simulink model "SizingFlightModel"  (R2024b)
settings: Solver=VariableStepAuto  StartTime=0.0  StopTime=50  RelTol=1e-3
values from neighbouring files (symbols this model uses):
  gamma = 1.4    [PotentialOrificeSize.m]    (also in runSizingSim.m = 1.23; sizingSweep.m = 1.23)
  isp = 215    [runSizingSim.m]    (also in sizingSweep.m)
  M = readmatrix(filename, 'NumHeaderLines', 1)    [STEPFNC_ODE_THRUST.m]    (also in runSizingSim.m = 0.0288; sizingSweep.m = 0.0288)
  m_0 = m_payload + 1.15 * m_fuel    (= 25.75)    [runSizingSim.m]    (also in sizingSweep.m = m_payload + 1.15 * m_fuel)
  m_fuel = 5.0    (= 5)    [runSizingSim.m]
  mdot = mdot_limit    (= 0.4)    [PotentialOrificeSize.m]    (also in runSizingSim.m = 0.359302325581; sizingSweep.m = result_table.MassFlowRate_kgps)
  p_c = 520 * 6894.76    (= 3585275.2)    [runSizingSim.m]    (also in sizingSweep.m)
  r = 0.08    [runSizingSim.m]    (also in sizingPrep.m = 0.1016; sizingSweep.m; tankEquilibrium.m = 0.1016)
  T_c = 3200    [runSizingSim.m]    (also in sizingSweep.m)
libraries: simulink x2, aerolibatmos2 x2
settings Model: Creator=Nicholas Quillin  LastModifiedBy=Nicholas Quillin

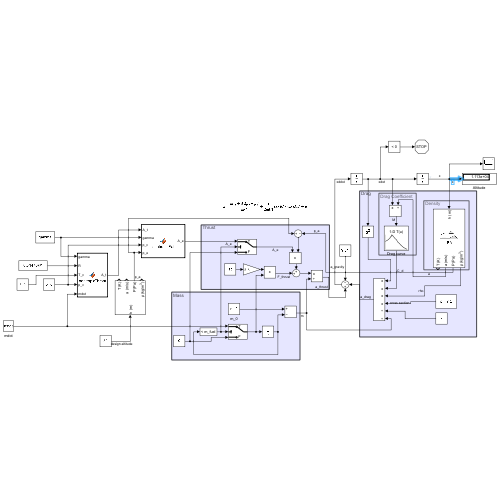
[thumbnail: Simulink's stored preview of the top-level diagram]
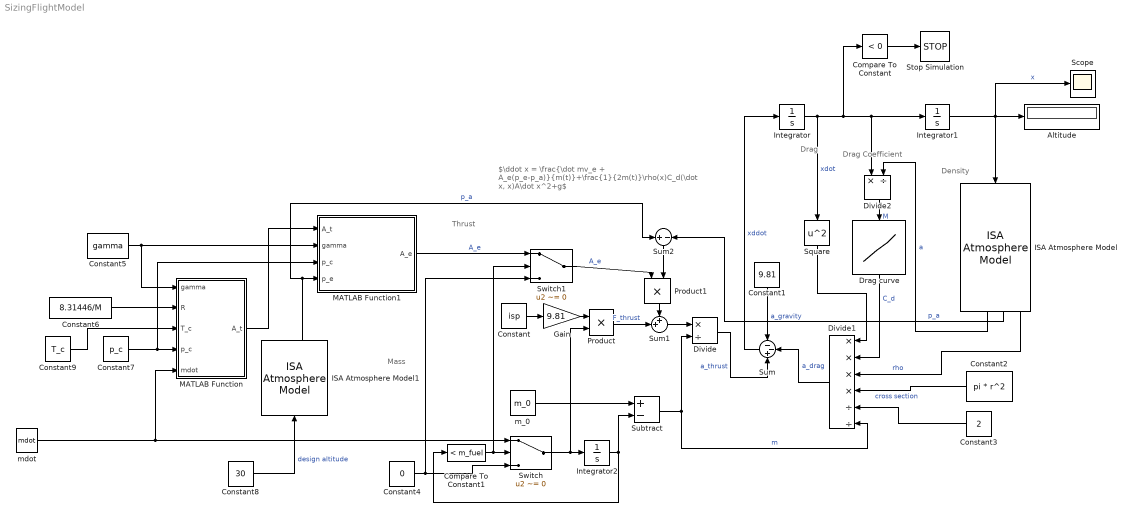
== system SizingFlightModel ==
  note: $\ddot x = \frac{\dot mv_e + A_e(p_e-p_a)}{m(t)}+\frac{1}{2m(t)}\rho(x)C_d(\dot x, x)A\dot x^2+g$
  note: Density
  note: Drag Coefficient
  note: Mass
  note: Thrust
  note: Drag
  Altitude : Display
  Compare To Constant : simulink/Logic and Bit Operations/Compare To Constant  relop=<  const=0  OutDataTypeStr=boolean
  Compare To Constant1 : simulink/Logic and Bit Operations/Compare To Constant  relop=<  const=m_fuel  OutDataTypeStr=boolean
  Constant : Constant  Value=isp
  Constant1 : Constant  Value=9.81
  Constant2 : Constant  Value=pi * r^2
  Constant3 : Constant  Value=2
  Constant4 : Constant  Value=0
  Constant5 : Constant  Value=gamma
  Constant6 : Constant  Value=8.31446/M
  Constant7 : Constant  Value=p_c
  Constant8 : Constant  Value=30
  Constant9 : Constant  Value=T_c
  Divide : Product  Inputs=*/
  Divide1 : Product  Inputs=****//
  Divide2 : Product  Inputs=*/
  Drag curve : Lookup_n-D  NumberOfTableDimensions=1  BreakpointsForDimension1=[0.2 0.4 0.6 0.8 0.9 0.975 1.0 1.025 1.05 1.1 1.2 1.4 1.6 1.8 2.0 2.2 2.4 2.6 2.8 3.0]  Table=[0.52 0.534 0.559 0.592 0.612 0.628 0.649 0.651 0.655 0.648 0.629 0.590 0.549 0.508 0.472 0.442 0.414 0.390 0.371 0.355]  InterpMethod=Linear Lagrange  InternalRulePriority=Speed  RndMeth=Simplest
  Gain : Gain  Gain=9.81
  ISA Atmosphere Model : aerolibatmos2/ISA Atmosphere Model  useExtended=off  action=Warning  custom=off  viscosityOut=off  g=9.80665  gamma=1.4  R=287.0531  L=0.0065  h_trop=11000  h_strat=20000  rho0=1.225  P0=101325  T0=288.15  h0=0  S=110.4  Tref=273.15  muref=1.716e-5
  ISA Atmosphere Model1 : aerolibatmos2/ISA Atmosphere Model  useExtended=off  action=Warning  custom=off  viscosityOut=off  g=9.80665  gamma=1.4  R=287.0531  L=0.0065  h_trop=11000  h_strat=20000  rho0=1.225  P0=101325  T0=288.15  h0=0  S=110.4  Tref=273.15  muref=1.716e-5
  Integrator : Integrator
  Integrator1 : Integrator
  Integrator2 : Integrator
  MATLAB Function : MATLAB Function  TreatAsAtomicUnit=on
  MATLAB Function1 : MATLAB Function  TreatAsAtomicUnit=on
  Product : Product
  Product1 : Product
  Scope : Scope
  Square : Math  Operator=square
  Stop Simulation : Stop
  Subtract : Sum  Inputs=+-
  Sum : Sum  Inputs=--+
  Sum1 : Sum  Inputs=++|
  Sum2 : Sum  Inputs=+-
  Switch : Switch  Criteria=u2 ~= 0  Threshold=m_fuel  SaturateOnIntegerOverflow=off  InputSameDT=off
  Switch1 : Switch  Criteria=u2 ~= 0  Threshold=m_fuel  SaturateOnIntegerOverflow=off  InputSameDT=off
  m_0 : Constant  Value=m_0
  mdot : Constant  Value=mdot
  wires:
  Sum/1 -> Integrator/1  "xddot"
  Integrator/1 -> Square/1, Compare To Constant/1, Divide2/1, Integrator1/1  "xdot"
  Integrator1/1 -> Altitude/1, Scope/1, ISA Atmosphere Model/1  "x"
  m_0/1 -> Subtract/1
  Integrator2/1 -> Subtract/2, Compare To Constant1/1
  Subtract/1 -> Divide1/6, Divide/2  "m"
  Drag curve/1 -> Divide1/2  "C_d"
  Switch/1 -> Product/2, Integrator2/1
  mdot/1 -> MATLAB Function/5(mdot), Switch/1
  Divide/1 -> Sum/3  "a_thrust"
  Divide1/1 -> Sum/2  "a_drag"
  Constant1/1 -> Sum/1  "a_gravity"
  Square/1 -> Divide1/1
  ISA Atmosphere Model/4 -> Divide1/3  "rho"
  Constant2/1 -> Divide1/4  "cross section"
  Constant3/1 -> Divide1/5
  Divide2/1 -> Drag curve/1  "M"
  ISA Atmosphere Model/2 -> Divide2/2  "a"
  Compare To Constant/1 -> Stop Simulation/1
  Compare To Constant1/1 -> Switch1/2, Switch/2
  Constant4/1 -> Switch1/3, Switch/3
  MATLAB Function1/1(A_e) -> Switch1/1  "A_e"
  Product/1 -> Sum1/2  "F_thrust"
  Sum1/1 -> Divide/1
  Product1/1 -> Sum1/1
  Switch1/1 -> Product1/1  "A_e"
  Sum2/1 -> Product1/2
  ISA Atmosphere Model/3 -> Sum2/2  "p_a"
  Constant/1 -> Gain/1
  Gain/1 -> Product/1
  MATLAB Function/1(A_t) -> MATLAB Function1/1(A_t)
  Constant7/1 -> MATLAB Function1/3(p_c), MATLAB Function/4(p_c)
  ISA Atmosphere Model1/3 -> Sum2/1, MATLAB Function1/4(p_e)  "p_a"
  Constant5/1 -> MATLAB Function/1(gamma), MATLAB Function1/2(gamma)
  Constant6/1 -> MATLAB Function/2(R)
  Constant8/1 -> ISA Atmosphere Model1/1  "design altitude"
  Constant9/1 -> MATLAB Function/3(T_c)

== matlab function SizingFlightModel/MATLAB Function1 ==
  data: A_t input; gamma input; A_e output; p_c input; p_e input
function A_e = isentropicExit(A_t, gamma, p_c, p_e)
A_e = A_t * (2/(gamma+1))^(1/(gamma-1)) * (p_c/p_e)^(1/gamma)...
    * sqrt(((gamma-1)/(gamma+1)*(1-(p_e/p_c)^((gamma-1)/gamma)))^-1)

== matlab function SizingFlightModel/MATLAB Function ==
  data: gamma input; A_t output; R input; T_c input; p_c input; mdot input
function A_t = isentropicThroat(gamma, R, T_c, p_c, mdot)
A_t = mdot * sqrt(gamma*R*T_c) / p_c / gamma / sqrt((2/(gamma+1))^((gamma+1)/(gamma-1)))
